simulink model "week3_Problem1"  (R2020b)
settings: Solver=VariableStepAuto  StartTime=0.0  StopTime=200  RelTol=1e-3
settings Model: Creator=Akshay A H  LastModifiedBy=Akshay A H

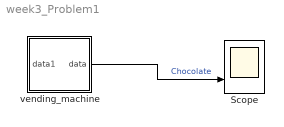
== system week3_Problem1 ==
  Scope : Scope  NumInputPorts=2
  vending_machine : Stateflow chart  TreatAsAtomicUnit=on
  wires:
  vending_machine/1(data) -> Scope/2  "Chocolate"

== stateflow chart week3_Problem1/vending_machine ==
  state Got_0
  state Got_Nickel
  state Got_Dime
  (default) -> Got_0
  Got_0 -> Got_Nickel [order 1] : [data1==1]{data=0}
  Got_Nickel -> Got_0 [order 1] : [data1==2]{data=1}
  Got_Dime -> Got_0 [order 2] : [data1==1]{data=1}
  Got_0 -> Got_Dime [order 2] : [data1==2]{data=0}
  Got_Nickel -> Got_Dime [order 2] : [data1==1]{data=0}
  Got_Dime -> Got_Nickel [order 1] : [data1==2]{data=1}
  data: data output; data1 input
